simulink model "pb6"  (R2020b)
settings: Solver=VariableStepAuto  StartTime=0.0  StopTime=10.0  MaxStep=.001  RelTol=1e-3
settings Model: Creator=SAGAR  LastModifiedBy=SAGAR

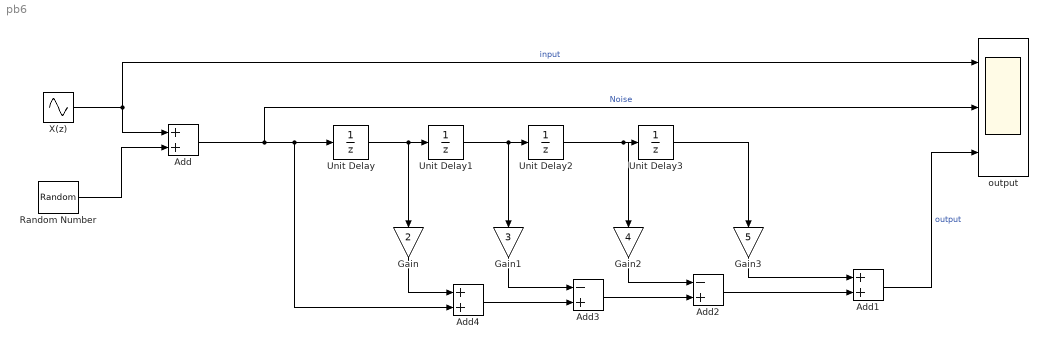
== system pb6 ==
  Add : Sum
  Add1 : Sum
  Add2 : Sum  Inputs=-+
  Add3 : Sum  Inputs=-+
  Add4 : Sum
  Gain : Gain  Gain=2
  Gain1 : Gain  Gain=3
  Gain2 : Gain  Gain=4
  Gain3 : Gain  Gain=5
  Random Number : RandomNumber  SampleTime=0.1
  Unit Delay{,1..3} (4 alike) : UnitDelay  SampleTime=-1  HasFrameUpgradeWarning=on
  X(z) : Sin  SampleTime=0
  output : Scope  NumInputPorts=3
  wires:
  Unit Delay/1 -> Gain/1, Unit Delay1/1
  Unit Delay1/1 -> Gain1/1, Unit Delay2/1
  Unit Delay2/1 -> Gain2/1, Unit Delay3/1
  Add/1 -> output/2, Add4/2, Unit Delay/1  "Noise"
  Unit Delay3/1 -> Gain3/1
  Gain/1 -> Add4/1
  Gain1/1 -> Add3/1
  Gain2/1 -> Add2/1
  Gain3/1 -> Add1/1
  Add4/1 -> Add3/2
  Add3/1 -> Add2/2
  Add2/1 -> Add1/2
  Add1/1 -> output/3  "output"
  X(z)/1 -> Add/1, output/1  "input"
  Random Number/1 -> Add/2
